simulink model "modelo_motor_P2"  (R2022b)
settings: Solver=VariableStepAuto  StartTime=0.0  StopTime=T_end  RelTol=1e-3
values from neighbouring files (symbols this model uses):
  Gz = c2d(G,Tm)    [lanza_P2.m]
  k_nl = 1.55    [lanza_P2.m]
  m = 3    [lanza_P2.m]
  Tm = 0.01    [lanza_P2.m]
  Vel_sat = 9.74    [lanza_P2.m]
  Volt_dead = 0.5    [lanza_P2.m]
libraries: cstblocks x2, dspsrcs4 x2
settings Model: Creator=jvalls  LastModifiedBy=pablo
settings SolverCC: AlgebraicLoopSolver=TrustRegion
settings DataIOCC: ReturnWorkspaceOutputs=off
settings OptimizationCC: LifeSpan=inf
settings DebuggingCC: UnconnectedInputMsg=warning  UnconnectedOutputMsg=warning  UnconnectedLineMsg=warning  SFExecutionAtInitializationDiag=none  SFMachineParentedDataDiag=warning  ArithmeticOperatorsInVariantConditions=warning
settings ModelReferenceCC: EnableRefExpFcnMdlSchedulingChecks=on
settings SFSimCC: SimUseLocalCustomCode=off  CustomCodeUndefinedFunction=UseInterfaceOnly
settings RTWCC: RTWUseLocalCustomCode=off  DLArmComputeVersion=19.05
settings CodeAppCC: StateflowObjectComments=on

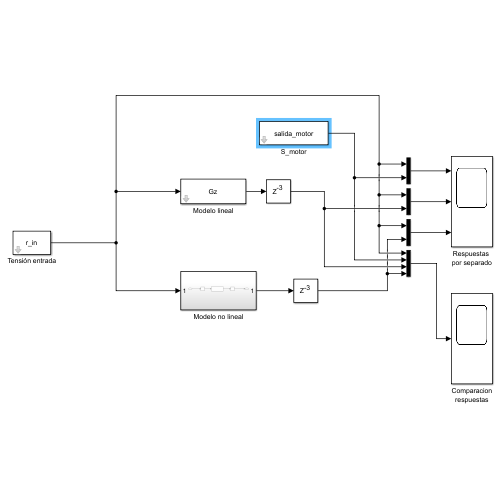
[thumbnail: Simulink's stored preview of the top-level diagram]
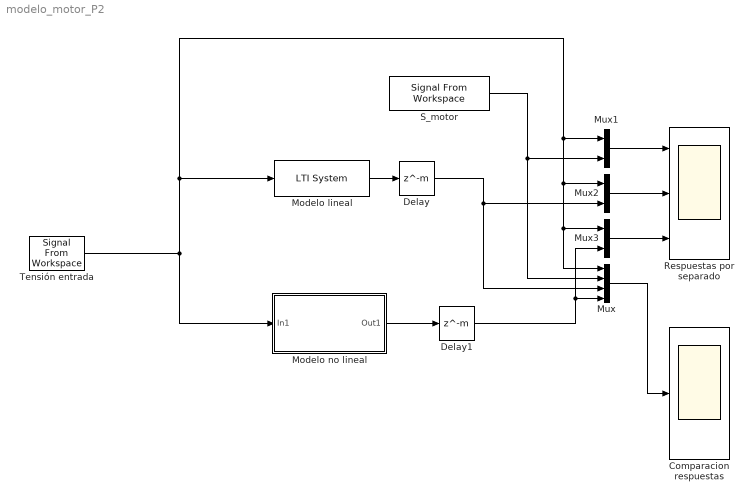
== system modelo_motor_P2 ==
  Comparacion respuestas : Scope
  Delay : Delay  DelayLength=m  InitialCondition=0
  Delay1 : Delay  DelayLength=m  InitialCondition=0
  Modelo lineal : cstblocks/LTI System  sys=Gz  IC=[]
  Modelo no lineal : Subsystem
  Mux : Mux
  Mux1 : Mux  Inputs=2
  Mux2 : Mux  Inputs=2
  Mux3 : Mux  Inputs=2
  Respuestas por separado : Scope  NumInputPorts=3
  S_motor : dspsrcs4/Signal From Workspace  X=salida_motor  Ts=Tm  nsamps=1  OutputAfterFinalValue=Setting to zero  ignoreOrWarnInputAndFrameLengths=off  OutputFrames=off
  Tensión entrada : dspsrcs4/Signal From Workspace  X=r_in  Ts=Tm  nsamps=1  OutputAfterFinalValue=Setting to zero  ignoreOrWarnInputAndFrameLengths=off  OutputFrames=off
  wires:
  Modelo lineal/1 -> Delay/1
  S_motor/1 -> Mux1/2, Mux/2
  Mux/1 -> Comparacion respuestas/1
  Mux1/1 -> Respuestas por separado/1
  Mux2/1 -> Respuestas por separado/2
  Mux3/1 -> Respuestas por separado/3
  Tensión entrada/1 -> Modelo no lineal/1(In1), Modelo lineal/1, Mux1/1, Mux2/1, Mux3/1, Mux/1
  Modelo no lineal/1(Out1) -> Delay1/1
  Delay/1 -> Mux2/2, Mux/3
  Delay1/1 -> Mux3/2, Mux/4

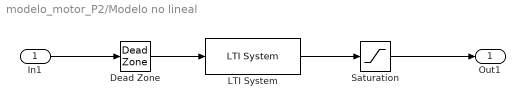
== system modelo_motor_P2/Modelo no lineal ==
  In1 : Inport
  "Dead Zone " : DeadZone  LowerValue=-Volt_dead  UpperValue=Volt_dead  SaturateOnIntegerOverflow=off
  "LTI System " : cstblocks/LTI System  sys=Gz*k_nl  IC=[]
  "Saturation " : Saturate  UpperLimit=Vel_sat  LowerLimit=-Vel_sat
  Out1 : Outport
  wires:
  "LTI System "/1 -> "Saturation "/1
  In1/1 -> "Dead Zone "/1
  "Saturation "/1 -> Out1/1
  "Dead Zone "/1 -> "LTI System "/1
